simulink subsystem "A313"  (R2022b)
settings: Solver=VariableStepAuto  StartTime=0.0  StopTime=10.0  RelTol=1e-3
settings Model: Creator=virgi  LastModifiedBy=virgi

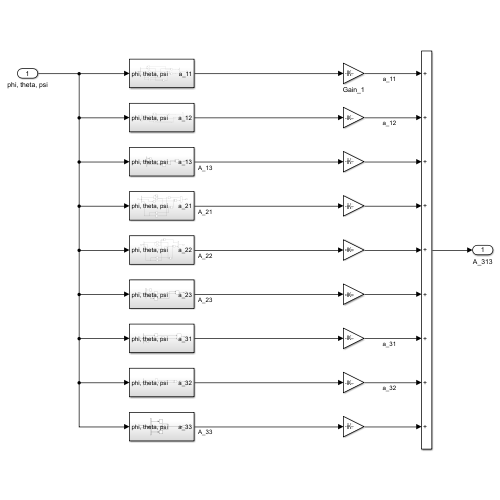
[thumbnail: Simulink's stored preview of the top-level diagram]
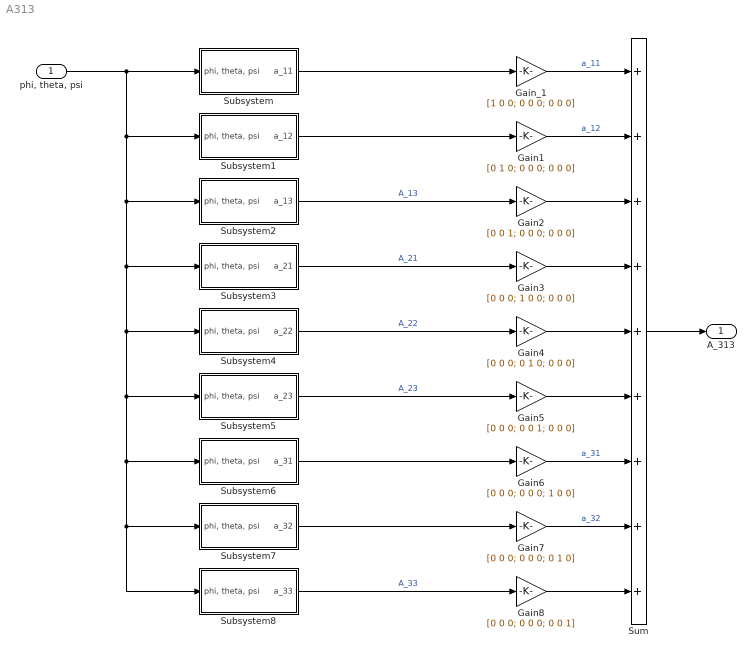
== system A313 ==
  "phi, theta, psi" : Inport
  Gain1 : Gain  Gain=[0 1 0; 0 0 0; 0 0 0]
  Gain2 : Gain  Gain=[0 0 1; 0 0 0; 0 0 0]
  Gain3 : Gain  Gain=[0 0 0; 1 0 0; 0 0 0]
  Gain4 : Gain  Gain=[0 0 0; 0 1 0; 0 0 0]
  Gain5 : Gain  Gain=[0 0 0; 0 0 1; 0 0 0]
  Gain6 : Gain  Gain=[0 0 0; 0 0 0; 1 0 0]
  Gain7 : Gain  Gain=[0 0 0; 0 0 0; 0 1 0]
  Gain8 : Gain  Gain=[0 0 0; 0 0 0; 0 0 1]
  Gain_1 : Gain  Gain=[1 0 0; 0 0 0; 0 0 0]
  Subsystem : Subsystem
  Subsystem1 : Subsystem
  Subsystem2 : Subsystem
  Subsystem3 : Subsystem
  Subsystem4 : Subsystem
  Subsystem5 : Subsystem
  Subsystem6 : Subsystem
  Subsystem7 : Subsystem
  Subsystem8 : Subsystem
  Sum : Sum  Inputs=+++++++++
  A_313 : Outport
  wires:
  Subsystem7/1(a_32) -> Gain7/1
  Subsystem2/1(a_13) -> Gain2/1  "A_13"
  Subsystem6/1(a_31) -> Gain6/1
  Gain5/1 -> Sum/6
  Gain7/1 -> Sum/8  "a_32"
  Sum/1 -> A_313/1
  Gain_1/1 -> Sum/1  "a_11"
  Subsystem5/1(a_23) -> Gain5/1  "A_23"
  Subsystem8/1(a_33) -> Gain8/1  "A_33"
  Gain3/1 -> Sum/4
  Gain4/1 -> Sum/5
  Gain2/1 -> Sum/3
  Subsystem/1(a_11) -> Gain_1/1
  Subsystem3/1(a_21) -> Gain3/1  "A_21"
  Subsystem4/1(a_22) -> Gain4/1  "A_22"
  Subsystem1/1(a_12) -> Gain1/1
  "phi, theta, psi"/1 -> Subsystem1/1("phi, theta, psi"), Subsystem2/1("phi, theta, psi"), Subsystem3/1("phi, theta, psi"), Subsystem4/1("phi, theta, psi"), Subsystem5/1("phi, theta, psi"), Subsystem6/1("phi, theta, psi"), Subsystem7/1("phi, theta, psi"), Subsystem8/1("phi, theta, psi"), Subsystem/1("phi, theta, psi")
  Gain6/1 -> Sum/7  "a_31"
  Gain8/1 -> Sum/9
  Gain1/1 -> Sum/2  "a_12"

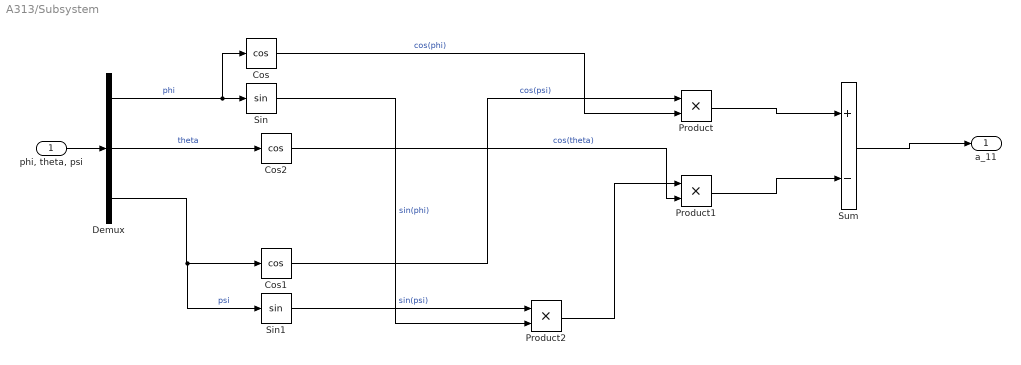
== system A313/Subsystem ==
  "phi, theta, psi" : Inport
  Cos : Trigonometry  Operator=cos
  Cos1 : Trigonometry  Operator=cos
  Cos2 : Trigonometry  Operator=cos
  Demux : Demux  Outputs=3
  Product : Product
  Product1 : Product
  Product2 : Product
  Sin : Trigonometry
  Sin1 : Trigonometry
  Sum : Sum  Inputs=+-
  a_11 : Outport
  wires:
  "phi, theta, psi"/1 -> Demux/1
  Demux/1 -> Sin/1, Cos/1  "phi"
  Demux/2 -> Cos2/1  "theta"
  Demux/3 -> Sin1/1, Cos1/1  "psi"
  Cos/1 -> Product/2  "cos(phi)"
  Sin/1 -> Product2/2  "sin(phi)"
  Sin1/1 -> Product2/1  "sin(psi)"
  Sum/1 -> a_11/1
  Cos1/1 -> Product/1  "cos(psi)"
  Product/1 -> Sum/1
  Product2/1 -> Product1/1
  Cos2/1 -> Product1/2  "cos(theta)"
  Product1/1 -> Sum/2

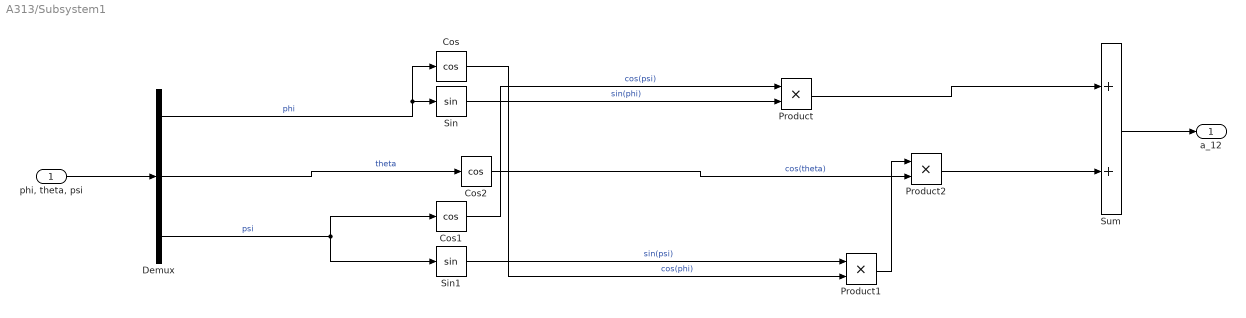
== system A313/Subsystem1 ==
  "phi, theta, psi" : Inport
  Cos : Trigonometry  Operator=cos
  Cos1 : Trigonometry  Operator=cos
  Cos2 : Trigonometry  Operator=cos
  Demux : Demux  Outputs=3
  Product : Product
  Product1 : Product
  Product2 : Product
  Sin : Trigonometry
  Sin1 : Trigonometry
  Sum : Sum
  a_12 : Outport
  wires:
  "phi, theta, psi"/1 -> Demux/1
  Demux/1 -> Cos/1, Sin/1  "phi"
  Cos2/1 -> Product2/2  "cos(theta)"
  Sin1/1 -> Product1/1  "sin(psi)"
  Cos1/1 -> Product/1  "cos(psi)"
  Sin/1 -> Product/2  "sin(phi)"
  Cos/1 -> Product1/2  "cos(phi)"
  Demux/3 -> Sin1/1, Cos1/1  "psi"
  Demux/2 -> Cos2/1  "theta"
  Sum/1 -> a_12/1
  Product1/1 -> Product2/1
  Product/1 -> Sum/1
  Product2/1 -> Sum/2

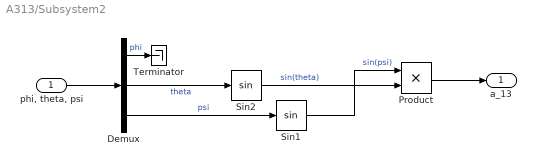
== system A313/Subsystem2 ==
  "phi, theta, psi" : Inport
  Demux : Demux  Outputs=3
  Product : Product
  Sin1 : Trigonometry
  Sin2 : Trigonometry
  Terminator : Terminator
  a_13 : Outport
  wires:
  "phi, theta, psi"/1 -> Demux/1
  Sin1/1 -> Product/1  "sin(psi)"
  Demux/2 -> Sin2/1  "theta"
  Sin2/1 -> Product/2  "sin(theta)"
  Demux/3 -> Sin1/1  "psi"
  Demux/1 -> Terminator/1  "phi"
  Product/1 -> a_13/1

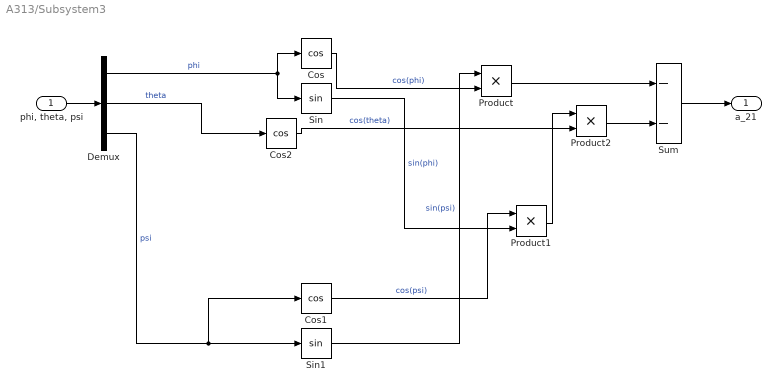
== system A313/Subsystem3 ==
  "phi, theta, psi" : Inport
  Cos : Trigonometry  Operator=cos
  Cos1 : Trigonometry  Operator=cos
  Cos2 : Trigonometry  Operator=cos
  Demux : Demux  Outputs=3
  Product : Product
  Product1 : Product
  Product2 : Product
  Sin : Trigonometry
  Sin1 : Trigonometry
  Sum : Sum  Inputs=--
  a_21 : Outport
  wires:
  "phi, theta, psi"/1 -> Demux/1
  Demux/1 -> Sin/1, Cos/1  "phi"
  Cos2/1 -> Product2/2  "cos(theta)"
  Sin1/1 -> Product/1  "sin(psi)"
  Cos1/1 -> Product1/1  "cos(psi)"
  Sin/1 -> Product1/2  "sin(phi)"
  Cos/1 -> Product/2  "cos(phi)"
  Demux/3 -> Cos1/1, Sin1/1  "psi"
  Demux/2 -> Cos2/1  "theta"
  Sum/1 -> a_21/1
  Product2/1 -> Sum/2
  Product1/1 -> Product2/1
  Product/1 -> Sum/1

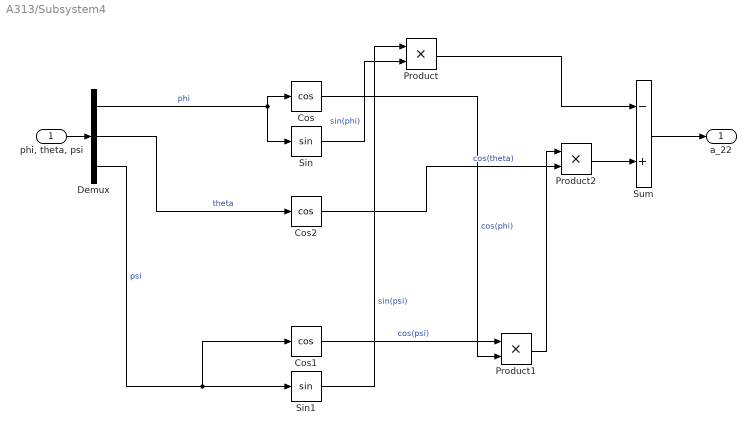
== system A313/Subsystem4 ==
  "phi, theta, psi" : Inport
  Cos : Trigonometry  Operator=cos
  Cos1 : Trigonometry  Operator=cos
  Cos2 : Trigonometry  Operator=cos
  Demux : Demux  Outputs=3
  Product : Product
  Product1 : Product
  Product2 : Product
  Sin : Trigonometry
  Sin1 : Trigonometry
  Sum : Sum  Inputs=-+
  a_22 : Outport
  wires:
  "phi, theta, psi"/1 -> Demux/1
  Demux/1 -> Sin/1, Cos/1  "phi"
  Cos2/1 -> Product2/2  "cos(theta)"
  Sin1/1 -> Product/1  "sin(psi)"
  Cos1/1 -> Product1/1  "cos(psi)"
  Sin/1 -> Product/2  "sin(phi)"
  Cos/1 -> Product1/2  "cos(phi)"
  Demux/3 -> Cos1/1, Sin1/1  "psi"
  Demux/2 -> Cos2/1  "theta"
  Sum/1 -> a_22/1
  Product2/1 -> Sum/2
  Product1/1 -> Product2/1
  Product/1 -> Sum/1

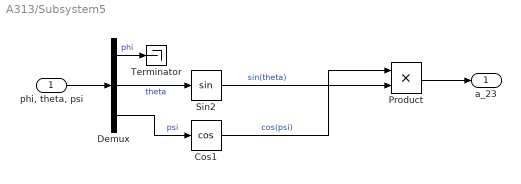
== system A313/Subsystem5 ==
  "phi, theta, psi" : Inport
  Cos1 : Trigonometry  Operator=cos
  Demux : Demux  Outputs=3
  Product : Product
  Sin2 : Trigonometry
  Terminator : Terminator
  a_23 : Outport
  wires:
  "phi, theta, psi"/1 -> Demux/1
  Cos1/1 -> Product/1  "cos(psi)"
  Demux/2 -> Sin2/1  "theta"
  Sin2/1 -> Product/2  "sin(theta)"
  Demux/3 -> Cos1/1  "psi"
  Demux/1 -> Terminator/1  "phi"
  Product/1 -> a_23/1

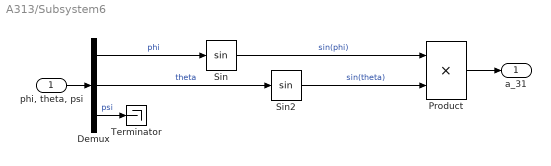
== system A313/Subsystem6 ==
  "phi, theta, psi" : Inport
  Demux : Demux  Outputs=3
  Product : Product
  Sin : Trigonometry
  Sin2 : Trigonometry
  Terminator : Terminator
  a_31 : Outport
  wires:
  "phi, theta, psi"/1 -> Demux/1
  Demux/1 -> Sin/1  "phi"
  Sin/1 -> Product/1  "sin(phi)"
  Demux/2 -> Sin2/1  "theta"
  Sin2/1 -> Product/2  "sin(theta)"
  Demux/3 -> Terminator/1  "psi"
  Product/1 -> a_31/1

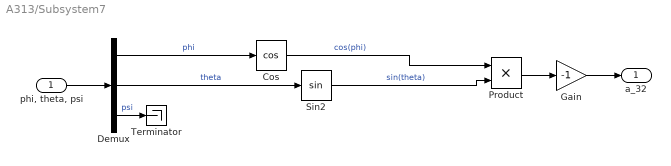
== system A313/Subsystem7 ==
  "phi, theta, psi" : Inport
  Cos : Trigonometry  Operator=cos
  Demux : Demux  Outputs=3
  Gain : Gain  Gain=-1
  Product : Product
  Sin2 : Trigonometry
  Terminator : Terminator
  a_32 : Outport
  wires:
  "phi, theta, psi"/1 -> Demux/1
  Demux/1 -> Cos/1  "phi"
  Demux/2 -> Sin2/1  "theta"
  Sin2/1 -> Product/2  "sin(theta)"
  Cos/1 -> Product/1  "cos(phi)"
  Demux/3 -> Terminator/1  "psi"
  Product/1 -> Gain/1
  Gain/1 -> a_32/1

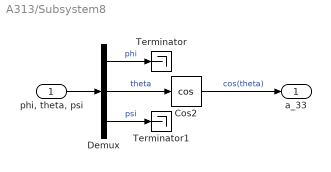
== system A313/Subsystem8 ==
  "phi, theta, psi" : Inport
  Cos2 : Trigonometry  Operator=cos
  Demux : Demux  Outputs=3
  Terminator : Terminator
  Terminator1 : Terminator
  a_33 : Outport
  wires:
  "phi, theta, psi"/1 -> Demux/1
  Cos2/1 -> a_33/1  "cos(theta)"
  Demux/2 -> Cos2/1  "theta"
  Demux/3 -> Terminator1/1  "psi"
  Demux/1 -> Terminator/1  "phi"
